simulink model "fsfb1"  (R2019b)
settings: Solver=VariableStepAuto  StartTime=0.0  StopTime=10.0  RelTol=1e-3
libraries: robotlib x4
settings Model: Creator=aaryansh  LastModifiedBy=aaryansh

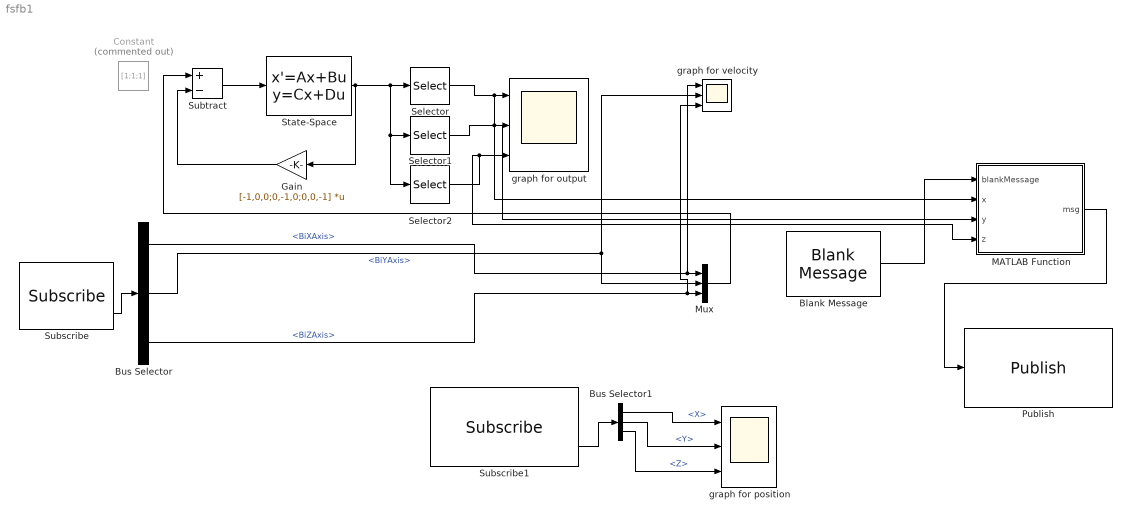
== system fsfb1 ==
  Blank Message : robotlib/Blank Message  messageClass=Message  entityType=std_msgs/Float64MultiArray  messageType=std_msgs/Float64MultiArray  SampleTime=inf
      settings: SourceProductName=ROS Toolbox
  Bus Selector : BusSelector  OutputSignals=BiXAxis,BiYAxis,BiZAxis
  Bus Selector1 : BusSelector  OutputSignals=Position.X,Position.Y,Position.Z
  Constant : Constant  Commented=on  Value=[1;1;1]  VectorParams1D=off
  Gain : Gain  Gain=[-1,0,0;0,-1,0;0,0,-1]  Multiplication=Matrix(K*u) (u vector)
  MATLAB Function : MATLAB Function  TreatAsAtomicUnit=on
  Mux : Mux  Inputs=3
  Publish : robotlib/Publish  topicSource=Select from ROS network  topic=/g500/thrusters_input  messageType=std_msgs/Float64MultiArray  messageQueueLength=1
      settings: SourceProductName=ROS Toolbox
  Selector : Selector  InputPortWidth=3  IndexOptions=Index vector (dialog)  Indices=1  OutputSizes=1
  Selector1 : Selector  InputPortWidth=3  IndexOptions=Index vector (dialog)  Indices=2  OutputSizes=1
  Selector2 : Selector  InputPortWidth=3  IndexOptions=Index vector (dialog)  Indices=3  OutputSizes=1
  State-Space : StateSpace  A=[0,0,0;0,0,0;0,0,0]  B=[1,0,0;0,1,0;0,0,1]  C=[1,0,0;0,1,0;0,0,1]  D=[0,0,0;0,0,0;0,0,0]  InitialCondition=[0.25;1.507;3.9]
  Subscribe : robotlib/Subscribe  topicSource=Select from ROS network  topic=/g500/dvl  messageType=underwater_sensor_msgs/DVL  sampleTime=-1  messageQueueLength=1
      settings: SourceProductName=ROS Toolbox
  Subscribe1 : robotlib/Subscribe  topicSource=Select from ROS network  topic=/g500/pose  messageType=geometry_msgs/Pose  sampleTime=-1  messageQueueLength=1
      settings: SourceProductName=ROS Toolbox
  Subtract : Sum  Inputs=+-
  graph for output : Scope  NumInputPorts=3
  graph for position : Scope  NumInputPorts=3
  graph for velocity : Scope  NumInputPorts=3
  wires:
  Subtract/1 -> State-Space/1
  State-Space/1 -> Selector1/1, Selector2/1, Selector/1, Gain/1
  Gain/1 -> Subtract/2
  Selector/1 -> MATLAB Function/2(x), graph for output/1
  Selector1/1 -> MATLAB Function/3(y), graph for output/2
  Selector2/1 -> graph for output/3, MATLAB Function/4(z)
  Subscribe/2 -> Bus Selector/1
  Bus Selector/1 -> graph for velocity/1, Mux/1  "<BiXAxis>"
  Bus Selector/2 -> graph for velocity/2, Mux/2  "<BiYAxis>"
  Bus Selector/3 -> graph for velocity/3, Mux/3  "<BiZAxis>"
  Subscribe1/2 -> Bus Selector1/1
  Bus Selector1/1 -> graph for position/1  "<X>"
  Bus Selector1/2 -> graph for position/2  "<Y>"
  Bus Selector1/3 -> graph for position/3  "<Z>"
  Mux/1 -> Subtract/1
  Blank Message/1 -> MATLAB Function/1(blankMessage)
  MATLAB Function/1(msg) -> Publish/1

== matlab function fsfb1/MATLAB Function ==
  data: blankMessage input; msg output Bus: SL_Bus_fsfb1_std_msgs_Float64MultiArray; x input; y input; z input
function msg=thrustersMap(blankMessage,x,y,z)
msg=blankMessage;

msg.Data(1)=-y;
msg.Data(2)=-y;
msg.Data(3)=-z;
msg.Data(4)=-z;
msg.Data(5)=-x;

msg.Data_SL_Info.CurrentLength=uint32(5);
